simulink model "Q1_sim2"  (R2023b)
settings: Solver=VariableStepAuto  StartTime=0.0  StopTime=1.2  RelTol=1e-3
libraries: simulink x1
settings Model: Creator=avikd  LastModifiedBy=avikd

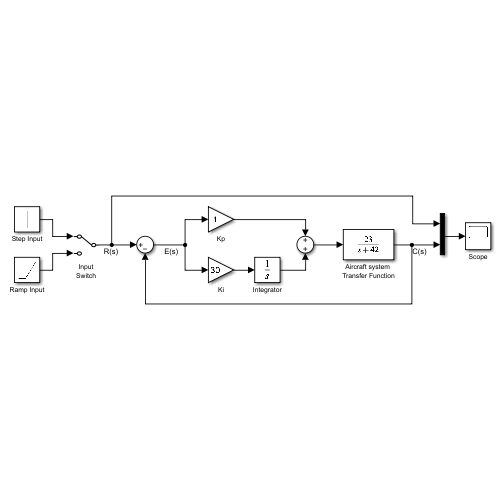
[thumbnail: Simulink's stored preview of the top-level diagram]
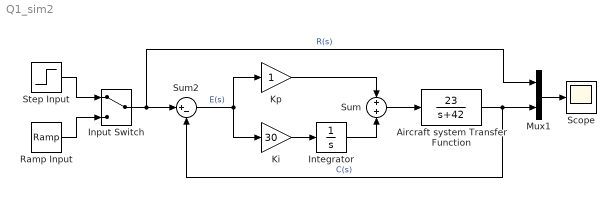
== system Q1_sim2 ==
  Aircraft system Transfer Function : TransferFcn  Numerator=[23]  Denominator=[1 42]
  Input Switch : ManualSwitch
  Integrator : Integrator
  Ki : Gain  Gain=30
  Kp : Gain
  Mux1 : Mux  Inputs=2
  Ramp Input : simulink/Sources/Ramp  slope=1  start=0  InitialOutput=0
  Scope : Scope
  Step Input : Step  Time=0  SampleTime=0
  Sum : Sum
  Sum2 : Sum  Inputs=|+-
  wires:
  Aircraft system Transfer Function/1 -> Mux1/2, Sum2/2  "C(s)"
  Step Input/1 -> Input Switch/1
  Sum2/1 -> Ki/1, Kp/1  "E(s)"
  Ramp Input/1 -> Input Switch/2
  Mux1/1 -> Scope/1
  Input Switch/1 -> Mux1/1, Sum2/1  "R(s)"
  Sum/1 -> Aircraft system Transfer Function/1
  Ki/1 -> Integrator/1
  Kp/1 -> Sum/1
  Integrator/1 -> Sum/2
